simulink model "CM012A_FordT3McuCfg"  (R2013b)
settings: Solver=FixedStepDiscrete  SolverMode=SingleTasking  StartTime=0.0  StopTime=2  FixedStep=0.00005  RelTol=1e-3
values from neighbouring files (symbols this model uses):
  BATTVLTGSCAGFAC_ULS_F32 = DataDict.Constant    [CM012A_FordT3McuCfg_DataDict.m]
  BATTVLTGSWD1SCAGFAC_ULS_F32 = DataDict.Constant    [CM012A_FordT3McuCfg_DataDict.m]
  CHRGPMPDIAGSCAGFAC_ULS_F32 = DataDict.Constant    [CM012A_FordT3McuCfg_DataDict.m]
  MOTAG2MEAS_ECU1OFFS_MOTREV_F32 = DataDict.Constant    [CM012A_FordT3McuCfg_DataDict.m]
  MOTAG2MEAS_ECU2OFFS_MOTREV_F32 = DataDict.Constant    [CM012A_FordT3McuCfg_DataDict.m]
  PWRDISCNCTSWTDIAGSCAGFAC_ULS_F32 = DataDict.Constant    [CM012A_FordT3McuCfg_DataDict.m]
undefined symbols (not defined in the file or in its folder): HwAgSnsrTyp1, sigbuilder_block
libraries: CM012A_FordT3McuCfg_ModelLibrary x114, simulink x37, NxtrLim x34
(part 4 of 4)

== system CM012A_FordT3McuCfg/FordT3McuCfg/FordT3McuCfgInit3/Wait for ADC Conversion to Complete/GetTiSpan1MicroSec32bit ==
  RefTmr : Inport
  CopyRight2 : Subsystem  Description=|  mask(Copyright Information){none=on}
      | Copyright info block.                                               
      |                                                                     
      | Place copyright information at the top of every subsystem in design.
      mask prompts: none "No parameters"
      mask help: Place copyright information at the top of every subsystem in design.
      mask Display:
      | NxtrConf = 'Nexteer Confidential';
      | 
      | sys = bdroot; %handle for the current model ("system")
      | first = get_param(sys,'Created');
      | first = first(end-3:end);  %year is last four digits
      | 
      | last = get_param(sys,'LastModifiedDate');
      | if isempty(last)
      |     last = datestr(now,'yyyy');
      | else
      |     last = last(end-3:end);
      | end
      | 
      | if strcmp(first,last)
      |     fprintf('%s -- Copyright %s Nexteer',NxtrConf,first)
      | else
      |     fprintf('%s -- %s%s- %s Nexteer',NxtrConf,char(169),first,last)
      | end
  Ground : Ground
  Terminator : Terminator
  TiSpan : Outport
  wires:
  Ground/1 -> TiSpan/1
  RefTmr/1 -> Terminator/1

== system CM012A_FordT3McuCfg/FordT3McuCfg/FordT3McuCfgInit4/Process Initial Adc1/CopyRight2 ==

== system CM012A_FordT3McuCfg/FordT3McuCfg/FordT3McuCfgInit5/If Action Subsystem/CopyRight2 ==

== system CM012A_FordT3McuCfg/FordT3McuCfg/FordT3McuCfgInit5/If Action Subsystem3/CopyRight2 ==

== system CM012A_FordT3McuCfg/FordT3McuCfg/FordT3McuCfgPer3/Adc0Faild Processing/CopyRight2 ==

== system CM012A_FordT3McuCfg/FordT3McuCfg/FordT3McuCfgPer3/Adc1Faild Processing/CopyRight2 ==

== system CM012A_FordT3McuCfg/FordT3McuCfg/FordT3McuCfgInit3/Wait for ADC Conversion to Complete/GetRefTmr1MicroSec32bit/CopyRight2 ==

== system CM012A_FordT3McuCfg/FordT3McuCfg/FordT3McuCfgInit3/Wait for ADC Conversion to Complete/GetTiSpan1MicroSec32bit/CopyRight2 ==
